simulink model "shoukongkalman"  (R2024b)
settings: Solver=FixedStepAuto  StartTime=0.0  StopTime=10.0  FixedStep=1  RelTol=1e-3
settings Model: Creator=54238  LastModifiedBy=54238

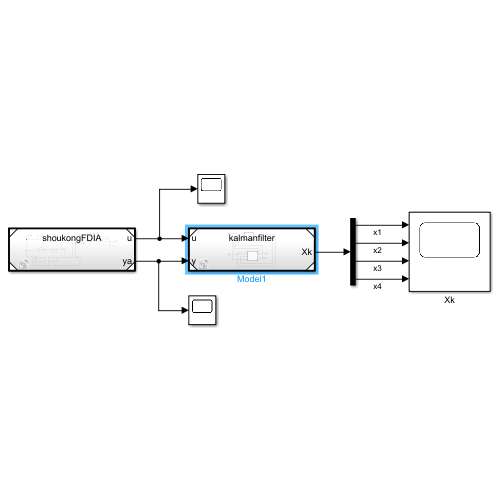
[thumbnail: Simulink's stored preview of the top-level diagram]
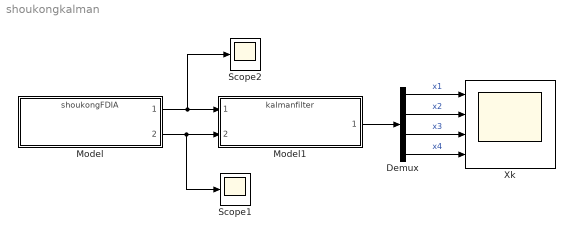
== system shoukongkalman ==
  Demux : Demux
  Model : ModelReference  ModelNameDialog=shoukongFDIA.slx  SimulationMode=Normal  ModelReferenceVersion=1.19
  Model1 : ModelReference  ModelNameDialog=kalmanfilter.slx  SimulationMode=Normal  ModelReferenceVersion=1.8
  Scope1 : Scope
  Scope2 : Scope
  Xk : Scope  NumInputPorts=4
  wires:
  Model/1 -> Scope2/1, Model1/1
  Model/2 -> Scope1/1, Model1/2
  Model1/1 -> Demux/1
  Demux/1 -> Xk/1  "x1"
  Demux/2 -> Xk/2  "x2"
  Demux/3 -> Xk/3  "x3"
  Demux/4 -> Xk/4  "x4"
